simulink model "dynamics"  (R2016b)
settings: Solver=ode23  StartTime=0.0  StopTime=inf  RelTol=1e-3
values from neighbouring files (symbols this model uses):
  A = [-1 1;0 -2]    [PIO_init.m]
  B = [0;1]    [PIO_init.m]
  C = eye(2)    [PIO_init.m]
  X_0 = zeros(2,1)    [PIO_init.m]
settings Model: Creator=samnazari  LastModifiedBy=samnazari

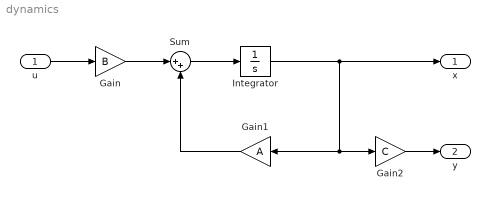
== system dynamics ==
  u : Inport
  Gain : Gain  Gain=B
  Gain1 : Gain  Gain=A
  Gain2 : Gain  Gain=C
  Integrator : Integrator  InitialCondition=X_0
  Sum : Sum  Inputs=|++
  x : Outport
  y : Outport  Port=2
  wires:
  u/1 -> Gain/1
  Gain/1 -> Sum/1
  Gain1/1 -> Sum/2
  Sum/1 -> Integrator/1
  Integrator/1 -> Gain2/1, Gain1/1, x/1
  Gain2/1 -> y/1
